simulink model "P2_0D_model_parametrized"  (R2023a)
settings: Solver=ode4  StartTime=0.0  StopTime=inf  FixedStep=Ts  RelTol=1e-3
model workspace (MAT data in the model file):
  Ts : Simulink.Parameter (value not decoded)
undefined symbols (not defined in the file or in its folder): data, HR, left_ventricle_R_wall, MLAP, MRAP, openloop
libraries: Vessel x42, simulink x2
(part 2 of 2)

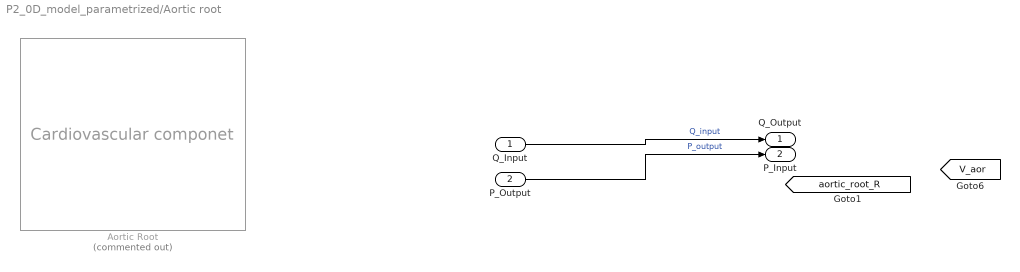
== system P2_0D_model_parametrized/Aortic root ==
  Q_Input : Inport
  P_Output : Inport  Port=2
  Aortic Root : Vessel/Cardiovascular componet  Commented=on  choice=Vessel compartment (L-non-inverted element)  control=None  Y_control=Systemic Arteries  l=aortic_root_l0  r=aortic_root_r0  h=aortic_root_h  n=aortic_root_n  P0=aortic_root_P0  Y=Y_aorta  SI=0  V_tot=V_tot  p_th_on_off=on
      link override "Capillaries (L-non-inverted-element)/ ": GotoTag=pupo
      settings: SourceProductName=CVM
  "Q_Output " : Outport
  "P_Input " : Outport  Port=2
  tag scope: V_aor=global, aortic_root_R=global
  wires:
  P_Output/1 -> "P_Input "/1  "P_output"
  Q_Input/1 -> "Q_Output "/1  "Q_input"

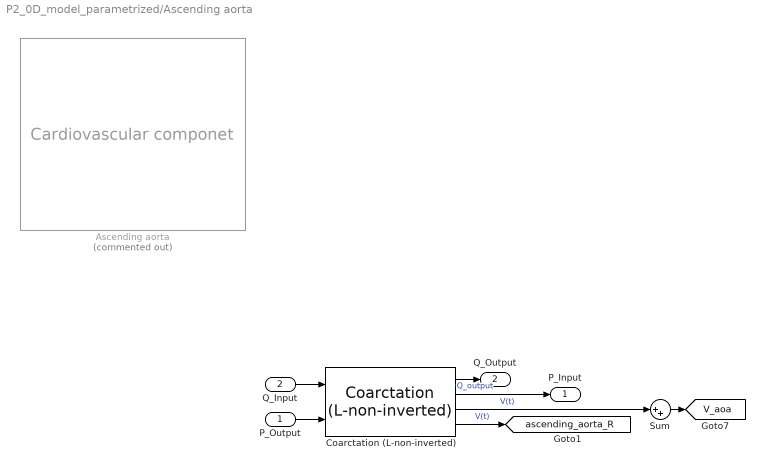
== system P2_0D_model_parametrized/Ascending aorta ==
  P_Output : Inport
  Q_Input : Inport  Port=2
  Ascending aorta : Vessel/Cardiovascular componet  Commented=on  choice=Vessel compartment (L-non-inverted element)  control=None  Y_control=Systemic Arteries  l=ascending_aorta_l0  r=ascending_aorta_r0  h=ascending_aorta_h  n=ascending_aorta_n  P0=ascending_aorta_P0  Y=Y_aorta  SI=0  V_tot=V_tot  p_th_on_off=on
      link override "Capillaries (L-non-inverted-element)/ ": GotoTag=pupo
      settings: SourceProductName=CVM
  Coarctation (L-non-inverted) : Vessel/Coarctation (L-non-inverted)  l=data.vessels{1, 1}.vessel_length  SI=data.vessels{1, 1}.zero_d_element_values.stenosis_coefficient  L0=data.vessels{1, 1}.zero_d_element_values.L  P0=100  Y=Y_aorta  Y_control=Systemic Arteries
      settings: SourceProductName=CVM
  Sum : Sum  Inputs=|++
  "P_Input " : Outport
  "Q_Output " : Outport  Port=2
  tag scope: V_aoa=global, ascending_aorta_R=global
  wires:
  P_Output/1 -> Coarctation (L-non-inverted)/2
  Q_Input/1 -> Coarctation (L-non-inverted)/1
  Coarctation (L-non-inverted)/1 -> "Q_Output "/1  "Q_output"
  Coarctation (L-non-inverted)/3 -> Sum/1  "V(t)"
  Coarctation (L-non-inverted)/4 -> [ascending_aorta_R]  "V(t)"
  Sum/1 -> [V_aoa]
  Coarctation (L-non-inverted)/2 -> "P_Input "/1

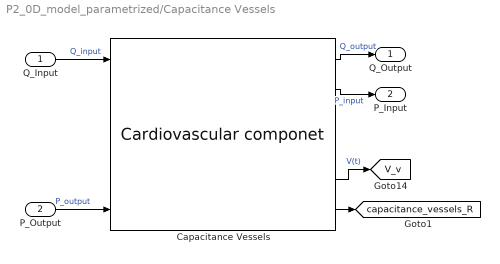
== system P2_0D_model_parametrized/Capacitance Vessels ==
  Q_Input : Inport
  P_Output : Inport  Port=2
  Capacitance Vessels : Vessel/Cardiovascular componet  choice=Vessel compartment (L-non-inverted element)  control=UVV control  Y_control=Systemic Veins  l=capacitance_vessels_l0  r=capacitance_vessels_r0  h=capacitance_vessels_h  n=capacitance_vessels_n  P0=capacitance_vessels_P0  Y=Y_systemic_veins  SI=0  V_tot=V_tot  p_th_on_off=off
      link override "Capillaries (L-non-inverted-element)/ ": GotoTag=pupo
      link override Vessel (L-non-inverted) /Constant1: Value=V0
      link override Vessel (L-non-inverted) Volume control/Constant1: Value=V0
      settings: SourceProductName=CVM
  "Q_Output " : Outport
  "P_Input " : Outport  Port=2
  tag scope: V_v=global, capacitance_vessels_R=global
  wires:
  Capacitance Vessels/5 -> [V_v]  "V(t)"
  Capacitance Vessels/2 -> "P_Input "/1  "P_input"
  P_Output/1 -> Capacitance Vessels/4  "P_output"
  Q_Input/1 -> Capacitance Vessels/1  "Q_input"
  Capacitance Vessels/1 -> "Q_Output "/1  "Q_output"
  Capacitance Vessels/6 -> [capacitance_vessels_R]

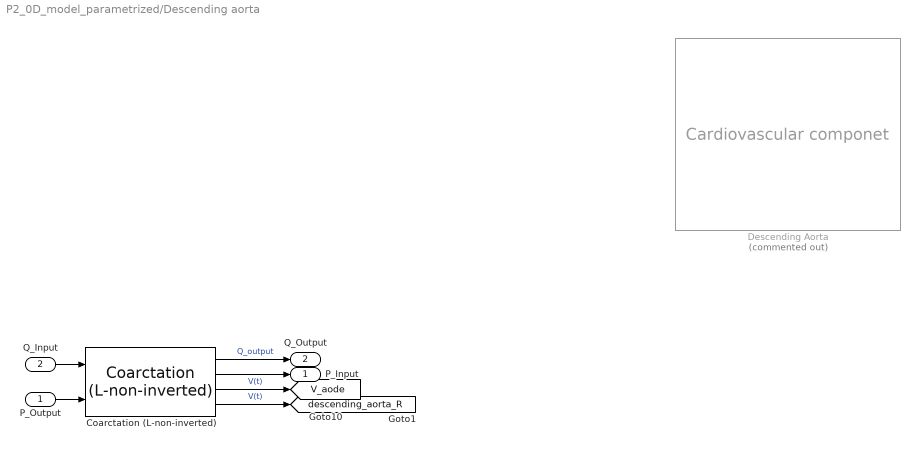
== system P2_0D_model_parametrized/Descending aorta ==
  P_Output : Inport
  Q_Input : Inport  Port=2
  Coarctation (L-non-inverted) : Vessel/Coarctation (L-non-inverted)  l=data.vessels{9,1}.vessel_length  SI=data.vessels{9, 1}.zero_d_element_values.stenosis_coefficient  L0=data.vessels{9, 1}.zero_d_element_values.L  P0=100  Y=Y_aorta  Y_control=Systemic Arteries
      settings: SourceProductName=CVM
  Descending Aorta : Vessel/Cardiovascular componet  Commented=on  choice=Vessel compartment (L-non-inverted element)  control=None  Y_control=Systemic Arteries  l=descending_aorta_l0  r=descending_aorta_r0  h=descending_aorta_h  n=descending_aorta_n  P0=descending_aorta_P0  Y=Y_aorta  SI=0  V_tot=V_tot  p_th_on_off=on
      link override "Capillaries (L-non-inverted-element)/ ": GotoTag=pupo
      settings: SourceProductName=CVM
  "P_Input " : Outport
  "Q_Output " : Outport  Port=2
  tag scope: V_aode=global, descending_aorta_R=global
  wires:
  Coarctation (L-non-inverted)/2 -> "P_Input "/1
  Q_Input/1 -> Coarctation (L-non-inverted)/1
  P_Output/1 -> Coarctation (L-non-inverted)/2
  Coarctation (L-non-inverted)/1 -> "Q_Output "/1  "Q_output"
  Coarctation (L-non-inverted)/3 -> [V_aode]  "V(t)"
  Coarctation (L-non-inverted)/4 -> [descending_aorta_R]  "V(t)"

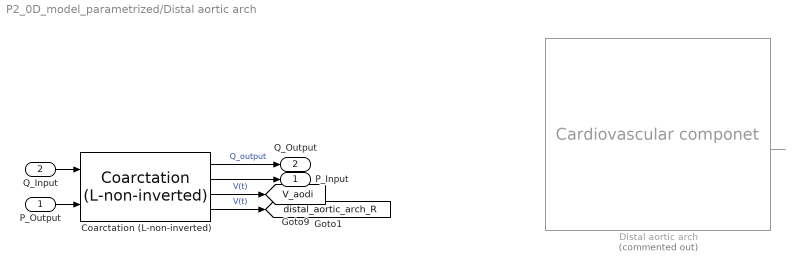
== system P2_0D_model_parametrized/Distal aortic arch ==
  P_Output : Inport
  Q_Input : Inport  Port=2
  Coarctation (L-non-inverted) : Vessel/Coarctation (L-non-inverted)  l=data.vessels{8, 1}.vessel_length  SI=data.vessels{8, 1}.zero_d_element_values.stenosis_coefficient  L0=data.vessels{8, 1}.zero_d_element_values.L  P0=100  Y=Y_aorta  Y_control=Systemic Arteries
      settings: SourceProductName=CVM
  Distal aortic arch : Vessel/Cardiovascular componet  Commented=on  choice=Vessel compartment (L-non-inverted element)  control=None  Y_control=Systemic Arteries  l=distal_aortic_arch_l0  r=distal_aortic_arch_r0  h=distal_aortic_arch_h  n=distal_aortic_arch_n  P0=distal_aortic_arch_P0  Y=Y_aorta  SI=0  V_tot=V_tot  p_th_on_off=on
      link override "Capillaries (L-non-inverted-element)/ ": GotoTag=pupo
      settings: SourceProductName=CVM
  "P_Input " : Outport
  "Q_Output " : Outport  Port=2
  tag scope: V_aodi=global, distal_aortic_arch_R=global
  wires:
  Q_Input/1 -> Coarctation (L-non-inverted)/1
  P_Output/1 -> Coarctation (L-non-inverted)/2
  Distal aortic arch/4 -> ?
  Coarctation (L-non-inverted)/1 -> "Q_Output "/1  "Q_output"
  Coarctation (L-non-inverted)/2 -> "P_Input "/1
  Coarctation (L-non-inverted)/3 -> [V_aodi]  "V(t)"
  Coarctation (L-non-inverted)/4 -> [distal_aortic_arch_R]  "V(t)"

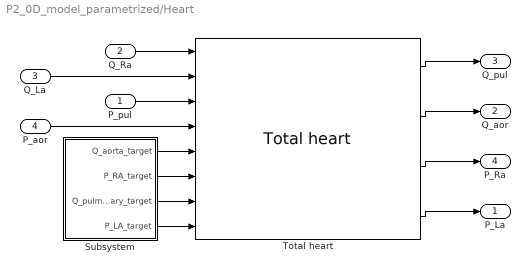
== system P2_0D_model_parametrized/Heart ==
  P_pul : Inport
  Q_Ra : Inport  Port=2
  Q_La : Inport  Port=3
  P_aor : Inport  Port=4
  Subsystem : Subsystem
  Total heart : Vessel/Total heart  BSA=BSA  T0=60/HR  R_lca=left_coronary_artery_R0  R_rca=right_coronary_artery_R0  p_septum_on_off=on  E_max_ra=right_atrium_E_max  E_max_rv=right_ventricle_E_max  E_max_la=left_atrium_E_max  E_max_lv=left_ventricle_E_max  E_min_ra=right_atrium_E_min  E_min_rv=right_ventricle_E_min  E_min_la=left_atrium_E_min  E_min_lv=left_ventricle_E_min  alpha1_ra=right_atrium_alpha1  alpha1_rv=right_ventricle_alpha1  alpha1_la=left_atrium_alpha1  alpha1_lv=left_ventricle_alpha1  alpha2_ra=right_atrium_alpha2  alpha2_rv=right_ventricle_alpha2  alpha2_la=left_atrium_alpha2  alpha2_lv=left_ventricle_alpha2  m1_ra=right_atrium_m1  m1_rv=right_ventricle_m1  m1_la=left_atrium_m1  m1_lv=left_ventricle_m1  m2_ra=right_atrium_m2  m2_rv=right_ventricle_m2  m2_la=left_atrium_m2  m2_lv=left_ventricle_m2  R_wall_ra=right_atrium_R_wall  R_wall_rv=right_ventricle_R_wall  R_wall_la=left_atrium_R_wall  R_wall_lv=left_ventricle_R_wall*1  t_delay_ra=right_atrium_t_delay  t_delay_rv=right_ventricle_t_delay  t_delay_la=left_atrium_t_delay  t_delay_lv=left_ventricle_t_delay  V_0_ra=right_atrium_V0  V_0_rv=right_ventricle_V0  V_0_la=left_atrium_V0  V_0_lv=left_ventricle_V0  v_o_ra=right_atrium_v0  v_o_rv=right_ventricle_v0  v_o_la=left_atrium_v0  v_o_lv=left_ventricle_v0  sigma_ra=right_atrium_sigma  sigma_rv=right_ventricle_sigma  sigma_la=left_atrium_sigma  sigma_lv=left_ventricle_sigma  V_max_ra=right_atrium_V_max  V_max_rv=right_ventricle_V_max  V_max_la=left_atrium_V_max  V_max_lv=left_ventricle_V_max  Q_max_ra=right_atrium_Q_max  Q_max_rv=right_ventricle_Q_max  Q_max_la=left_atrium_Q_max  Q_max_lv=left_ventricle_Q_max  A_ann_tri=tricuspid_valve_A_ann  A_ann_pul=pulmonary_valve_A_ann  A_ann_mit=mitral_valve_A_ann  A_ann_aor=aortic_valve_A_ann  K_vo_tri=tricuspid_valve_K_vo  K_vo_pul=pulmonary_valve_K_vo  K_vo_mit=mitral_valve_K_vo  K_vo_aor=aortic_valve_K_vo  K_vc_tri=tricuspid_valve_K_vc  K_vc_pul=pulmonary_valve_K_vc  K_vc_mit=mitral_valve_K_vc  K_vc_aor=aortic_valve_K_vc  M_st_tri=tricuspid_valve_M_st  M_st_pul=pulmonary_valve_M_st  M_st_mit=mitral_valve_M_st  M_st_aor=aortic_valve_M_st  M_rg_tri=tricuspid_valve_M_rg  M_rg_pul=pulmonary_valve_M_rg  M_rg_mit=mitral_valve_M_rg  M_rg_aor=aortic_valve_M_rg  DP_open_tri=tricuspid_valve_DP_open  DP_open_pul=pulmonary_valve_DP_open  DP_open_mit=mitral_valve_DP_open  DP_open_aor=aortic_valve_DP_open  DP_close_tri=tricuspid_valve_DP_close  DP_close_pul=pulmonary_valve_DP_close  DP_close_mit=mitral_valve_DP_close  DP_close_aor=aortic_valve_DP_close  P_pc_0=P_pc0  K_pc=K_pc  V_pc_0=V_pc  V_pe=PFV  phi_pc=phi_pc  E_sa_0=E_sa0  E_sv_0=E_sv0
      link override Aortic Valve/Saturation1: UpperLimit=100  LowerLimit=0.000
      link override Aortic Valve/Saturation2: UpperLimit=100
      link override Left Atrium: control=Left Atrium
      link override Mitral valve/Saturation1: LowerLimit=0.0000
      link override Pulmonary Valve/Saturation1: UpperLimit=100  LowerLimit=0.0000
      link override Right Atrium: control=Right Atrium
      link override Right Ventricle: control=Right Ventricle
      link override Tricuspid Valve/Saturation1: LowerLimit=0.0000
      link override Volume Control: V_tot_0=V_tot
      settings: SourceProductName=CVM
  P_La : Outport
  Q_aor : Outport  Port=2
  Q_pul : Outport  Port=3
  P_Ra : Outport  Port=4
  wires:
  Total heart/4 -> P_La/1
  Total heart/2 -> Q_aor/1
  Total heart/1 -> Q_pul/1
  Q_Ra/1 -> Total heart/1
  P_pul/1 -> Total heart/3
  Q_La/1 -> Total heart/2
  P_aor/1 -> Total heart/4
  Total heart/3 -> P_Ra/1
  Subsystem/1(Q_aorta_target) -> Total heart/5
  Subsystem/2(P_RA_target) -> Total heart/6
  Subsystem/3(Q_pulmonary_target) -> Total heart/7
  Subsystem/4(P_LA_target) -> Total heart/8

== system P2_0D_model_parametrized/Inferior Caval Vein ==
  Q_Input : Inport
  P_Output : Inport  Port=2
  Inferior Caval Vein : Vessel/Cardiovascular componet  choice=Vessel compartment (L-non-inverted element)  control=None  Y_control=Systemic Veins  l=inferior_caval_vein_l0  r=inferior_caval_vein_r0  h=inferior_caval_vein_h  n=inferior_caval_vein_n  P0=inferior_caval_vein_P0  Y=Y_systemic_veins  SI=0  V_tot=V_tot  p_th_on_off=off
      link override "Capillaries (L-non-inverted-element)/ ": GotoTag=pupo
      settings: SourceProductName=CVM
  "P_Input " : Outport
  "Q_Output " : Outport  Port=2
  tag scope: V_vci=global, inferior_caval_vein_R=global
  wires:
  Inferior Caval Vein/2 -> "P_Input "/1
  Inferior Caval Vein/5 -> [V_vci]
  P_Output/1 -> Inferior Caval Vein/4
  Inferior Caval Vein/1 -> "Q_Output "/1
  Q_Input/1 -> Inferior Caval Vein/1
  Inferior Caval Vein/6 -> [inferior_caval_vein_R]

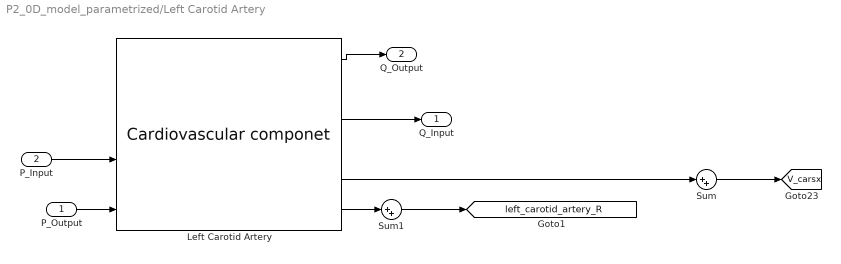
== system P2_0D_model_parametrized/Left Carotid Artery ==
  P_Output : Inport
  P_Input : Inport  Port=2
  Left Carotid Artery : Vessel/Cardiovascular componet  choice=Carotid Artery (L-non-inverted)  control=None  Y_control=Systemic Arteries  l=left_carotid_artery_l0  r=left_carotid_artery_r0  h=left_carotid_artery_h  n=left_carotid_artery_n  P0=left_carotid_artery_P0  Y=Y_aorta  SI=data.vessels{3, 1}.zero_d_element_values.stenosis_coefficient  V_tot=V_tot  p_th_on_off=off
      link override "Capillaries (L-non-inverted-element)/ ": GotoTag=pupo
      settings: SourceProductName=CVM
  Sum : Sum  Inputs=|++
  Sum1 : Sum  Inputs=|++
  Q_Input : Outport
  Q_Output : Outport  Port=2
  tag scope: V_carsx=global, left_carotid_artery_R=global
  wires:
  Left Carotid Artery/5 -> Sum/1
  P_Output/1 -> Left Carotid Artery/4
  Left Carotid Artery/1 -> Q_Output/1
  Sum/1 -> [V_carsx]
  P_Input/1 -> Left Carotid Artery/3
  Sum1/1 -> [left_carotid_artery_R]
  Left Carotid Artery/6 -> Sum1/1
  Left Carotid Artery/3 -> Q_Input/1

== system P2_0D_model_parametrized/Left Carotid Capillaries ==
  P_Output : Inport
  Q_Input : Inport  Port=2
  Left Carotid Capillaries : Vessel/Cardiovascular componet  choice=Capillary compartment (L-non-inverted element)  control=None  Y_control=Systemic Veins  l=left_carotid_capillaries_l0  r=left_carotid_capillaries_r0  h=left_carotid_capillaries_h  n=left_carotid_capillaries_n  P0=left_carotid_capillaries_P0  Y=Y_systemic_veins  SI=0  V_tot=V_tot  p_th_on_off=off
      link override "Capillaries (L-non-inverted-element)/ ": GotoTag=pupo
      settings: SourceProductName=CVM
  P_input : Outport
  Q_Out : Outport  Port=2
  tag scope: V_ccarsx=global, left_carotid_capillaries_R=global
  wires:
  Left Carotid Capillaries/5 -> [V_ccarsx]
  P_Output/1 -> Left Carotid Capillaries/4
  Left Carotid Capillaries/1 -> Q_Out/1
  Left Carotid Capillaries/2 -> P_input/1
  Q_Input/1 -> Left Carotid Capillaries/1
  Left Carotid Capillaries/6 -> [left_carotid_capillaries_R]

== system P2_0D_model_parametrized/Left Carotid Resistance Artery ==
  P_Output : Inport
  Q_Input1 : Inport  Port=2
  Left Carotid Resistance Artery : Vessel/Cardiovascular componet  choice=Vessel compartment (L-non-inverted element)  control=SVR control  Y_control=Systemic Arteries  l=left_carotid_resistance_artery_l0  r=left_carotid_resistance_artery_r0  h=left_carotid_resistance_artery_h  n=left_carotid_resistance_artery_n  P0=left_carotid_resistance_artery_P0  Y=Y_aorta  SI=0  V_tot=V_tot  p_th_on_off=off
      link override "Capillaries (L-non-inverted-element)/ ": GotoTag=pupo
      settings: SourceProductName=CVM
  P_input : Outport
  Q_Output : Outport  Port=2
  tag scope: V_rcarsx=global, left_carotid_resistance_artery_R=global
  wires:
  Left Carotid Resistance Artery/5 -> [V_rcarsx]
  Left Carotid Resistance Artery/1 -> Q_Output/1
  Q_Input1/1 -> Left Carotid Resistance Artery/1
  Left Carotid Resistance Artery/2 -> P_input/1
  P_Output/1 -> Left Carotid Resistance Artery/4
  Left Carotid Resistance Artery/6 -> [left_carotid_resistance_artery_R]

== system P2_0D_model_parametrized/Left Carotid Vein ==
  P_Output : Inport
  Q_Input : Inport  Port=2
  Left Carotid Vein : Vessel/Cardiovascular componet  choice=Vessel compartment (L-non-inverted element)  control=UVV control  Y_control=Systemic Veins  l=left_carotid_vein_l0  r=left_carotid_vein_r0  h=left_carotid_vein_h  n=left_carotid_vein_n  P0=left_carotid_vein_P0  Y=Y_systemic_veins  SI=0  V_tot=V_tot  p_th_on_off=off
      link override "Capillaries (L-non-inverted-element)/ ": GotoTag=pupo
      settings: SourceProductName=CVM
  "P_Input " : Outport
  "Q_Output " : Outport  Port=2
  tag scope: V_vcarsx=global, left_carotid_vein_R=global
  wires:
  Left Carotid Vein/5 -> [V_vcarsx]
  P_Output/1 -> Left Carotid Vein/4
  Left Carotid Vein/2 -> "P_Input "/1
  Q_Input/1 -> Left Carotid Vein/1
  Left Carotid Vein/1 -> "Q_Output "/1
  Left Carotid Vein/6 -> [left_carotid_vein_R]

== system P2_0D_model_parametrized/Peripheral Arteries ==
  P_Output : Inport
  Q_Input : Inport  Port=2
  Peripheral Arteries : Vessel/Cardiovascular componet  choice=Vessel compartment (L-non-inverted element)  control=SVR control  Y_control=Systemic Arteries  l=peripheral_arteries_l0  r=peripheral_arteries_r0  h=peripheral_arteries_h  n=peripheral_arteries_n  P0=peripheral_arteries_P0  Y=Y_aorta  SI=0  V_tot=V_tot  p_th_on_off=off
      link override "Capillaries (L-non-inverted-element)/ ": GotoTag=pupo
      settings: SourceProductName=CVM
  "P_Input " : Outport
  "Q_Output " : Outport  Port=2
  tag scope: V_a=global, peripheral_arteries_R=global
  wires:
  Peripheral Arteries/5 -> [V_a]
  Peripheral Arteries/2 -> "P_Input "/1
  P_Output/1 -> Peripheral Arteries/4
  Q_Input/1 -> Peripheral Arteries/1
  Peripheral Arteries/1 -> "Q_Output "/1
  Peripheral Arteries/6 -> [peripheral_arteries_R]

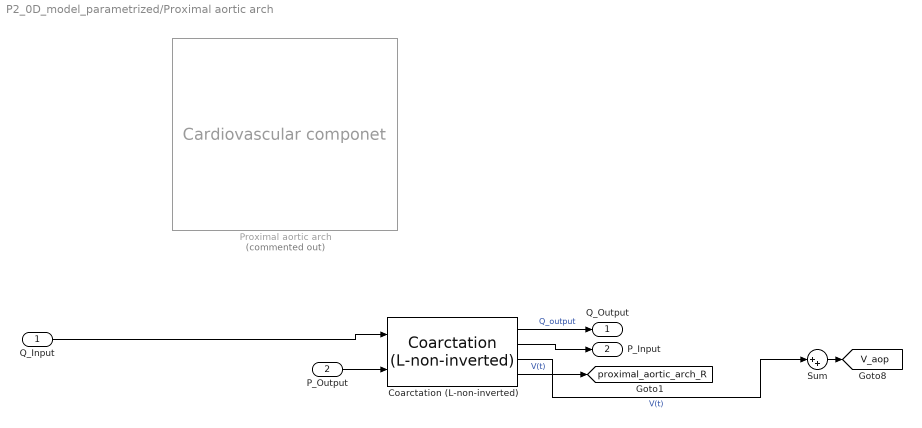
== system P2_0D_model_parametrized/Proximal aortic arch ==
  Q_Input : Inport
  P_Output : Inport  Port=2
  Coarctation (L-non-inverted) : Vessel/Coarctation (L-non-inverted)  l=data.vessels{7, 1}.vessel_length  SI=data.vessels{7, 1}.zero_d_element_values.stenosis_coefficient  L0=data.vessels{7, 1}.zero_d_element_values.L  P0=100  Y=Y_aorta  Y_control=Systemic Arteries
      settings: SourceProductName=CVM
  Proximal aortic arch : Vessel/Cardiovascular componet  Commented=on  choice=Vessel compartment (L-non-inverted element)  control=None  Y_control=Systemic Arteries  l=proximal_aortic_arch_l0  r=proximal_aortic_arch_r0  h=proximal_aortic_arch_h  n=proximal_aortic_arch_n  P0=proximal_aortic_arch_P0  Y=Y_aorta  SI=0  V_tot=V_tot  p_th_on_off=on
      link override "Capillaries (L-non-inverted-element)/ ": GotoTag=pupo
      settings: SourceProductName=CVM
  Sum : Sum  Inputs=|++
  "Q_Output " : Outport
  "P_Input " : Outport  Port=2
  tag scope: V_aop=global, proximal_aortic_arch_R=global
  wires:
  P_Output/1 -> Coarctation (L-non-inverted)/2
  Q_Input/1 -> Coarctation (L-non-inverted)/1
  Coarctation (L-non-inverted)/3 -> Sum/1  "V(t)"
  Coarctation (L-non-inverted)/4 -> [proximal_aortic_arch_R]  "V(t)"
  Coarctation (L-non-inverted)/1 -> "Q_Output "/1  "Q_output"
  Sum/1 -> [V_aop]
  Coarctation (L-non-inverted)/2 -> "P_Input "/1

== system P2_0D_model_parametrized/Pulmonary Arteries ==
  Q_Input : Inport
  P_Output : Inport  Port=2
  Pulmonary Arteries : Vessel/Cardiovascular componet  choice=Vessel compartment (L-non-inverted element)  control=None  Y_control=Pulmonary Arteries  l=pulmonary_arteries_l0  r=pulmonary_arteries_r0  h=pulmonary_arteries_h  n=pulmonary_arteries_n  P0=pulmonary_arteries_P0  Y=Y_pulmonary_arteries  SI=0  V_tot=V_tot  p_th_on_off=on
      link override "Capillaries (L-non-inverted-element)/ ": GotoTag=pupo
      settings: SourceProductName=CVM
  "Q_Output " : Outport
  "P_Input " : Outport  Port=2
  tag scope: V_pua=global, pulmonary_arteries_R=global
  wires:
  Pulmonary Arteries/5 -> [V_pua]
  Pulmonary Arteries/1 -> "Q_Output "/1
  Pulmonary Arteries/2 -> "P_Input "/1
  P_Output/1 -> Pulmonary Arteries/4
  Q_Input/1 -> Pulmonary Arteries/1
  Pulmonary Arteries/6 -> [pulmonary_arteries_R]

== system P2_0D_model_parametrized/Pulmonary Capillaries ==
  Q_Input : Inport
  P_Output : Inport  Port=2
  Pulmonary Capillaries : Vessel/Cardiovascular componet  choice=Capillary compartment (L-non-inverted element)  control=PVR control  Y_control=Pulmonary Veins  l=pulmonary_capillaries_l0  r=pulmonary_capillaries_r0  h=pulmonary_capillaries_h  n=pulmonary_capillaries_n  P0=pulmonary_capillaries_P0  Y=Y_pulmonary_veins  SI=0  V_tot=V_tot  p_th_on_off=on
      link override "Capillaries (L-non-inverted-element)/ ": GotoTag=pupo
      settings: SourceProductName=CVM
  "Q_Output " : Outport
  "P_Input " : Outport  Port=2
  tag scope: V_puc=global, pulmonary_capillaries_R=global
  wires:
  Pulmonary Capillaries/5 -> [V_puc]
  Pulmonary Capillaries/1 -> "Q_Output "/1
  Pulmonary Capillaries/2 -> "P_Input "/1
  P_Output/1 -> Pulmonary Capillaries/4
  Q_Input/1 -> Pulmonary Capillaries/1
  Pulmonary Capillaries/6 -> [pulmonary_capillaries_R]

== system P2_0D_model_parametrized/Pulmonary Resistance Arteries ==
  Q_Input : Inport
  P_Output : Inport  Port=2
  Pulmonary Resistance Arteries : Vessel/Cardiovascular componet  choice=Vessel compartment (L-non-inverted element)  control=PVR control  Y_control=Pulmonary Veins  l=pulmonary_resistance_arteries_l0  r=pulmonary_resistance_arteries_r0  h=pulmonary_resistance_arteries_h  n=pulmonary_resistance_arteries_n  P0=pulmonary_resistance_arteries_P0  Y=Y_pulmonary_veins  SI=0  V_tot=V_tot  p_th_on_off=on
      link override "Capillaries (L-non-inverted-element)/ ": GotoTag=pupo
      settings: SourceProductName=CVM
  "Q_Output " : Outport
  "P_Input " : Outport  Port=2
  tag scope: V_pur=global, pulmonary_resistance_arteries_R=global
  wires:
  Pulmonary Resistance Arteries/5 -> [V_pur]
  Pulmonary Resistance Arteries/2 -> "P_Input "/1
  P_Output/1 -> Pulmonary Resistance Arteries/4
  Pulmonary Resistance Arteries/1 -> "Q_Output "/1
  Q_Input/1 -> Pulmonary Resistance Arteries/1
  Pulmonary Resistance Arteries/6 -> [pulmonary_resistance_arteries_R]

== system P2_0D_model_parametrized/Pulmonary Small Veins ==
  Q_Input : Inport
  P_Output : Inport  Port=2
  Pulmonary Small Veins : Vessel/Cardiovascular componet  choice=Vessel compartment (L-non-inverted element)  control=PVR control  Y_control=Pulmonary Veins  l=pulmonary_small_veins_l0  r=pulmonary_small_veins_r0  h=pulmonary_small_veins_h  n=pulmonary_small_veins_n  P0=pulmonary_small_veins_P0  Y=Y_pulmonary_veins  SI=0  V_tot=V_tot  p_th_on_off=on
      link override "Capillaries (L-non-inverted-element)/ ": GotoTag=pupo
      settings: SourceProductName=CVM
  "Q_Output " : Outport
  "P_Input " : Outport  Port=2
  tag scope: V_pusv=global, pulmonary_small_veins_R=global
  wires:
  Pulmonary Small Veins/5 -> [V_pusv]
  Pulmonary Small Veins/1 -> "Q_Output "/1
  Q_Input/1 -> Pulmonary Small Veins/1
  Pulmonary Small Veins/2 -> "P_Input "/1
  P_Output/1 -> Pulmonary Small Veins/4
  Pulmonary Small Veins/6 -> [pulmonary_small_veins_R]

== system P2_0D_model_parametrized/Pulmonary Trunk ==
  P_Output : Inport
  Q_Input : Inport  Port=2
  Pulmonary Trunk : Vessel/Cardiovascular componet  choice=Vessel compartment (L-non-inverted element)  control=None  Y_control=Pulmonary Arteries  l=pulmonary_trunk_l0  r=pulmonary_trunk_r0  h=pulmonary_trunk_h  n=pulmonary_trunk_n  P0=pulmonary_trunk_P0  Y=Y_pulmonary_arteries  SI=0  V_tot=V_tot  p_th_on_off=on
      link override "Capillaries (L-non-inverted-element)/ ": GotoTag=pupo
      settings: SourceProductName=CVM
  "P_Input " : Outport
  "Q_Output " : Outport  Port=2
  tag scope: V_put=global, pulmonary_trunk_R=global
  wires:
  Pulmonary Trunk/2 -> "P_Input "/1
  Pulmonary Trunk/1 -> "Q_Output "/1
  P_Output/1 -> Pulmonary Trunk/4
  Pulmonary Trunk/5 -> [V_put]
  Q_Input/1 -> Pulmonary Trunk/1
  Pulmonary Trunk/6 -> [pulmonary_trunk_R]

== system P2_0D_model_parametrized/Pulmonary Veins ==
  Q_Input : Inport
  P_Output : Inport  Port=2
  Pulmonary Veins : Vessel/Cardiovascular componet  choice=Vessel compartment (L-non-inverted element)  control=None  Y_control=Pulmonary Veins  l=pulmonary_veins_l0  r=pulmonary_veins_r0  h=pulmonary_veins_h  n=pulmonary_veins_n  P0=pulmonary_veins_P0  Y=Y_pulmonary_veins  SI=0  V_tot=V_tot  p_th_on_off=on
      link override "Capillaries (L-non-inverted-element)/ ": GotoTag=pupo
      settings: SourceProductName=CVM
  "Q_Output " : Outport
  "P_Input " : Outport  Port=2
  tag scope: V_puv=global, pulmonary_veins_R=global
  wires:
  Pulmonary Veins/2 -> "P_Input "/1
  Pulmonary Veins/1 -> "Q_Output "/1
  Pulmonary Veins/5 -> [V_puv]
  P_Output/1 -> Pulmonary Veins/4
  Q_Input/1 -> Pulmonary Veins/1
  Pulmonary Veins/6 -> [pulmonary_veins_R]

== system P2_0D_model_parametrized/Resistance Arteries ==
  Q_Input : Inport
  P_Output : Inport  Port=2
  Resistance Arteries : Vessel/Cardiovascular componet  choice=Vessel compartment (L-non-inverted element)  control=SVR control  Y_control=Systemic Arteries  l=resistance_arteries_l0  r=resistance_arteries_r0  h=resistance_arteries_h  n=resistance_arteries_n  P0=resistance_arteries_P0  Y=Y_aorta  SI=0  V_tot=V_tot  p_th_on_off=off
      link override "Capillaries (L-non-inverted-element)/ ": GotoTag=pupo
      settings: SourceProductName=CVM
  "Q_Output " : Outport
  "P_Input " : Outport  Port=2
  tag scope: V_r=global, resistance_arteries_R=global
  wires:
  Resistance Arteries/5 -> [V_r]
  Resistance Arteries/1 -> "Q_Output "/1
  Resistance Arteries/2 -> "P_Input "/1
  P_Output/1 -> Resistance Arteries/4
  Q_Input/1 -> Resistance Arteries/1
  Resistance Arteries/6 -> [resistance_arteries_R]

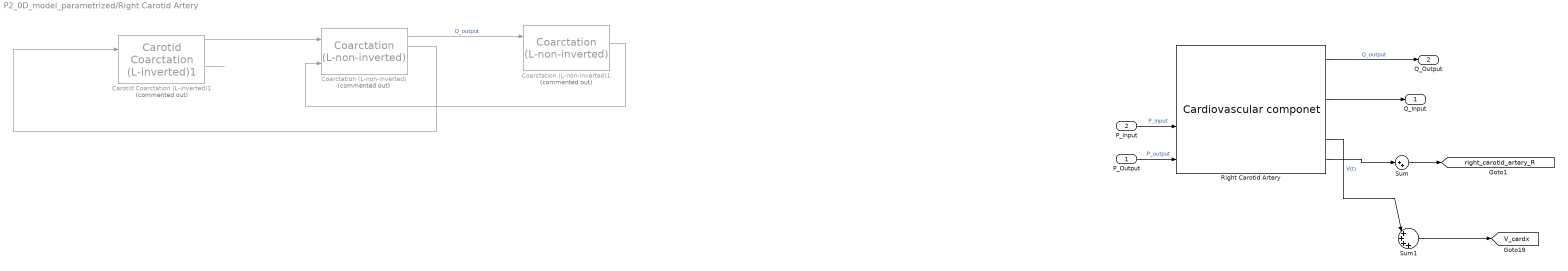
== system P2_0D_model_parametrized/Right Carotid Artery ==
  P_Output : Inport
  P_Input : Inport  Port=2
  Carotid Coarctation (L-inverted)1 : Vessel/Carotid Coarctation (L-inverted)1  Commented=on  l=data.vessels{10, 1}.vessel_length  SI=data.vessels{10, 1}.zero_d_element_values.stenosis_coefficient  L0=data.vessels{10, 1}.zero_d_element_values.L  P0=100  Y=Y_aorta  Y_control=Systemic arteries
      settings: SourceProductName=CVM
  Coarctation (L-non-inverted) : Vessel/Coarctation (L-non-inverted)  Commented=on  l=data.vessels{11, 1}.vessel_length  SI=data.vessels{11, 1}.zero_d_element_values.stenosis_coefficient  L0=data.vessels{11, 1}.zero_d_element_values.L  P0=100  Y=Y_aorta  Y_control=Systemic Arteries
      settings: SourceProductName=CVM
  Coarctation (L-non-inverted)1 : Vessel/Coarctation (L-non-inverted)  Commented=on  l=data.vessels{12, 1}.vessel_length  SI=data.vessels{12, 1}.zero_d_element_values.stenosis_coefficient  L0=data.vessels{12, 1}.zero_d_element_values.L  P0=100  Y=Y_aorta  Y_control=Systemic Arteries
      settings: SourceProductName=CVM
  Right Carotid Artery : Vessel/Cardiovascular componet  choice=Carotid Artery (L-non-inverted)  control=None  Y_control=Systemic Arteries  l=right_carotid_artery_l0  r=right_carotid_artery_r0  h=right_carotid_artery_h  n=right_carotid_artery_n  P0=right_carotid_artery_P0  Y=Y_aorta  SI=data.vessels{2, 1}.zero_d_element_values.stenosis_coefficient  V_tot=V_tot  p_th_on_off=off
      link override "Capillaries (L-non-inverted-element)/ ": GotoTag=pupo
      settings: SourceProductName=CVM
  Sum : Sum  Inputs=|++
  Sum1 : Sum  Inputs=|++++
  Q_Input : Outport
  Q_Output : Outport  Port=2
  tag scope: V_cardx=global, right_carotid_artery_R=global
  wires:
  P_Output/1 -> Right Carotid Artery/4  "P_output"
  Right Carotid Artery/1 -> Q_Output/1  "Q_output"
  Sum/1 -> [right_carotid_artery_R]
  Sum1/1 -> [V_cardx]
  Right Carotid Artery/3 -> Q_Input/1
  ? -> Carotid Coarctation (L-inverted)1/2  "P_input"
  Carotid Coarctation (L-inverted)1/1 -> Coarctation (L-non-inverted)/1
  Coarctation (L-non-inverted)/1 -> Coarctation (L-non-inverted)1/1  "Q_output"
  Coarctation (L-non-inverted)/2 -> Carotid Coarctation (L-inverted)1/1
  Coarctation (L-non-inverted)1/2 -> Coarctation (L-non-inverted)/2
  Carotid Coarctation (L-inverted)1/3 -> ?
  Right Carotid Artery/6 -> Sum/1
  Right Carotid Artery/5 -> Sum1/1  "V(t)"
  P_Input/1 -> Right Carotid Artery/3  "P_input"

== system P2_0D_model_parametrized/Right Carotid Capillaries ==
  P_Output : Inport
  Q_Input1 : Inport  Port=2
  Right Carotid Capillaries : Vessel/Cardiovascular componet  choice=Capillary compartment (L-non-inverted element)  control=None  Y_control=Systemic Veins  l=right_carotid_capillaries_l0  r=right_carotid_capillaries_r0  h=right_carotid_capillaries_h  n=right_carotid_capillaries_n  P0=right_carotid_capillaries_P0  Y=Y_systemic_veins  SI=0  V_tot=V_tot  p_th_on_off=off
      link override "Capillaries (L-non-inverted-element)/ ": GotoTag=pupo
      settings: SourceProductName=CVM
  P_input : Outport
  Q_Out : Outport  Port=2
  tag scope: V_ccardx=global, right_carotid_capillaries_R=global
  wires:
  Right Carotid Capillaries/5 -> [V_ccardx]
  Right Carotid Capillaries/1 -> Q_Out/1
  P_Output/1 -> Right Carotid Capillaries/4
  Q_Input1/1 -> Right Carotid Capillaries/1
  Right Carotid Capillaries/2 -> P_input/1
  Right Carotid Capillaries/6 -> [right_carotid_capillaries_R]

== system P2_0D_model_parametrized/Right Carotid Resistance Artery ==
  P_Output : Inport
  Q_Input1 : Inport  Port=2
  Right Carotid Resistance Artery : Vessel/Cardiovascular componet  choice=Vessel compartment (L-non-inverted element)  control=SVR control  Y_control=Systemic Arteries  l=right_carotid_resistance_artery_l0  r=right_carotid_resistance_artery_r0  h=right_carotid_resistance_artery_h  n=right_carotid_resistance_artery_n  P0=right_carotid_resistance_artery_P0  Y=Y_aorta  SI=0  V_tot=V_tot  p_th_on_off=off
      link override "Capillaries (L-non-inverted-element)/ ": GotoTag=pupo
      link override Vessel (L-inverted)/IC1: Value=0
      settings: SourceProductName=CVM
  P_input : Outport
  Q_Output : Outport  Port=2
  tag scope: V_rcardx=global, right_carotid_resistance_artery_R=global
  wires:
  Right Carotid Resistance Artery/5 -> [V_rcardx]
  P_Output/1 -> Right Carotid Resistance Artery/4
  Q_Input1/1 -> Right Carotid Resistance Artery/1
  Right Carotid Resistance Artery/2 -> P_input/1
  Right Carotid Resistance Artery/1 -> Q_Output/1
  Right Carotid Resistance Artery/6 -> [right_carotid_resistance_artery_R]

== system P2_0D_model_parametrized/Right Carotid Vein ==
  P_Output : Inport
  Q_Input : Inport  Port=2
  Right Carotid Vein : Vessel/Cardiovascular componet  choice=Vessel compartment (L-non-inverted element)  control=UVV control  Y_control=Systemic Veins  l=right_carotid_vein_l0  r=right_carotid_vein_r0  h=right_carotid_vein_h  n=right_carotid_vein_n  P0=right_carotid_vein_P0  Y=Y_systemic_veins  SI=0  V_tot=V_tot  p_th_on_off=off
      link override "Capillaries (L-non-inverted-element)/ ": GotoTag=pupo
      settings: SourceProductName=CVM
  "P_Input " : Outport
  "Q_Output " : Outport  Port=2
  tag scope: V_vcardx=global, right_carotid_vein_R=global
  wires:
  Right Carotid Vein/5 -> [V_vcardx]
  P_Output/1 -> Right Carotid Vein/4
  Right Carotid Vein/2 -> "P_Input "/1
  Q_Input/1 -> Right Carotid Vein/1
  Right Carotid Vein/1 -> "Q_Output "/1
  Right Carotid Vein/6 -> [right_carotid_vein_R]

== system P2_0D_model_parametrized/Superior Caval Vein ==
  Q_Input : Inport
  P_Output : Inport  Port=2
  Superior Caval Vein : Vessel/Cardiovascular componet  choice=Vessel compartment (L-non-inverted element)  control=None  Y_control=Systemic Veins  l=superior_caval_vein_l0  r=superior_caval_vein_r0  h=superior_caval_vein_h  n=superior_caval_vein_n  P0=superior_caval_vein_P0  Y=Y_systemic_veins  SI=0  V_tot=V_tot  p_th_on_off=off
      link override "Capillaries (L-non-inverted-element)/ ": GotoTag=pupo
      settings: SourceProductName=CVM
  "Q_Output " : Outport
  "P_Input " : Outport  Port=2
  tag scope: V_vcs=global, superior_caval_vein_R=global
  wires:
  Superior Caval Vein/2 -> "P_Input "/1
  Superior Caval Vein/1 -> "Q_Output "/1
  P_Output/1 -> Superior Caval Vein/4
  Superior Caval Vein/5 -> [V_vcs]
  Q_Input/1 -> Superior Caval Vein/1
  Superior Caval Vein/6 -> [superior_caval_vein_R]

== system P2_0D_model_parametrized/Systemic Capillaries  ==
  P_Output : Inport
  Q_Input : Inport  Port=2
  Systemic Capillaries : Vessel/Cardiovascular componet  choice=Capillary compartment (L-non-inverted element)  control=None  Y_control=Systemic Veins  l=systemic_capillaries_l0  r=systemic_capillaries_r0  h=systemic_capillaries_h  n=systemic_capillaries_n  P0=systemic_capillaries_P0  Y=Y_systemic_veins  SI=0  V_tot=V_tot  p_th_on_off=off
      link override "Capillaries (L-non-inverted-element)/ ": GotoTag=pupo
      settings: SourceProductName=CVM
  "P_Input " : Outport
  "Q_Output " : Outport  Port=2
  tag scope: V_c=global, systemic_capillaries_R=global
  wires:
  Systemic Capillaries/5 -> [V_c]  "V(t)"
  Systemic Capillaries/2 -> "P_Input "/1  "P_input"
  P_Output/1 -> Systemic Capillaries/4  "P_output"
  Q_Input/1 -> Systemic Capillaries/1  "Q_input"
  Systemic Capillaries/1 -> "Q_Output "/1  "Q_output"
  Systemic Capillaries/6 -> [systemic_capillaries_R]

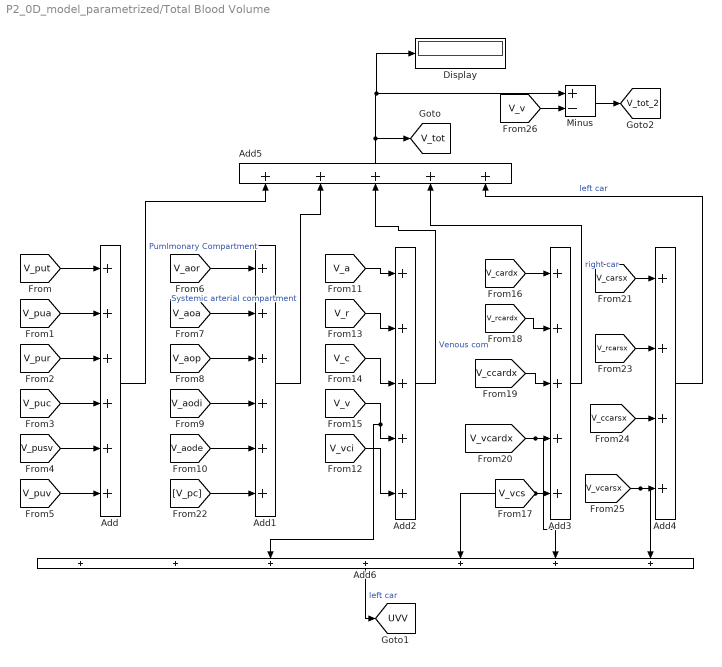
== system P2_0D_model_parametrized/Total Blood Volume ==
  Add : Sum  Inputs=++++++
  Add1 : Sum  Inputs=++++++
  Add2 : Sum  Inputs=+++++
  Add3 : Sum  Inputs=+++++
  Add4 : Sum  Inputs=++++
  Add5 : Sum  Inputs=+++++
  Add6 : Sum  Inputs=+++++++
  Display : Display
  Minus : Sum  Inputs=+-
  tag scope: UVV=global, V_tot=global, V_tot_2=global
  wires:
  [V_put] -> Add/1
  [V_pua] -> Add/2
  [V_pur] -> Add/3
  [V_puc] -> Add/4
  [V_pusv] -> Add/5
  [V_puv] -> Add/6
  [V_aor] -> Add1/1
  [V_aoa] -> Add1/2
  [V_aop] -> Add1/3
  [V_aodi] -> Add1/4
  [V_aode] -> Add1/5
  [V_a] -> Add2/1
  [V_r] -> Add2/2
  [V_c] -> Add2/3
  [V_v] -> Add6/3, Add2/4
  [V_vci] -> Add2/5
  [V_cardx] -> Add3/1
  [V_rcardx] -> Add3/2
  [V_ccardx] -> Add3/3
  [V_vcardx] -> Add6/6, Add3/4
  [V_vcs] -> Add6/5, Add3/5
  [V_carsx] -> Add4/1
  [V_rcarsx] -> Add4/2
  [V_ccarsx] -> Add4/3
  [V_pc] -> Add1/6
  Add/1 -> Add5/1  "Pumlmonary Compartment"
  Add1/1 -> Add5/2  "Systemic arterial compartment"
  Add2/1 -> Add5/3  "Venous com"
  Add3/1 -> Add5/4  "right car"
  Add4/1 -> Add5/5  "left car"
  Add5/1 -> [V_tot], Display/1, Minus/1
  [V_vcarsx] -> Add6/7, Add4/4
  Add6/1 -> [UVV]  "left car"
  Minus/1 -> [V_tot_2]
  [V_v] -> Minus/2

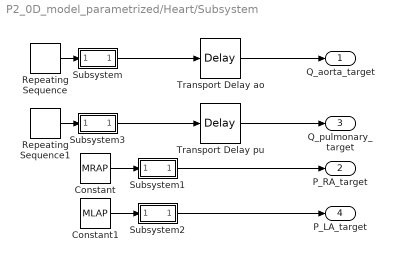
== system P2_0D_model_parametrized/Heart/Subsystem ==
  Constant : Constant  Value=MRAP
  Constant1 : Constant  Value=MLAP
  Repeating Sequence : simulink/Sources/Repeating Sequence  rep_seq_t=t  rep_seq_y=Q
  Repeating Sequence1 : simulink/Sources/Repeating Sequence  rep_seq_t=t  rep_seq_y=Q_p
  Subsystem : Subsystem
  Subsystem1 : Subsystem
  Subsystem2 : Subsystem
  Subsystem3 : Subsystem
  Transport Delay ao : TransportDelay  DelayTime=0
  Transport Delay pu : TransportDelay  DelayTime=0
  Q_aorta_target : Outport
  P_RA_target : Outport  Port=2
  Q_pulmonary_target : Outport  Port=3
  P_LA_target : Outport  Port=4
  wires:
  Repeating Sequence/1 -> Subsystem/1(In1)
  Constant/1 -> Subsystem1/1(In1)
  Constant1/1 -> Subsystem2/1(In1)
  Subsystem1/1(Out1) -> P_RA_target/1
  Subsystem2/1(Out1) -> P_LA_target/1
  Subsystem/1(Q_aorta_target) -> Transport Delay ao/1
  Repeating Sequence1/1 -> Subsystem3/1(In1)
  Subsystem3/1(Q_pulmonary_target) -> Transport Delay pu/1
  Transport Delay ao/1 -> Q_aorta_target/1
  Transport Delay pu/1 -> Q_pulmonary_target/1

== system P2_0D_model_parametrized/Heart/Subsystem/Subsystem ==
  In1 : Inport
  Constant2 : Constant  Value=openloop
  NaN : Constant  Value=NaN  OutDataTypeStr=Inherit: Inherit via back propagation
  Switch : Switch  Criteria=u2 > Threshold  SaturateOnIntegerOverflow=off  InputSameDT=off
  Q_aorta_target : Outport
  wires:
  In1/1 -> Switch/1
  Switch/1 -> Q_aorta_target/1
  Constant2/1 -> Switch/2
  NaN/1 -> Switch/3

== system P2_0D_model_parametrized/Heart/Subsystem/Subsystem1 ==
  In1 : Inport
  Constant2 : Constant  Value=openloop
  NaN : Constant  Value=NaN  OutDataTypeStr=Inherit: Inherit via back propagation
  Switch : Switch  Criteria=u2 > Threshold  SaturateOnIntegerOverflow=off  InputSameDT=off
  Out1 : Outport
  wires:
  NaN/1 -> Switch/3
  Constant2/1 -> Switch/2
  Switch/1 -> Out1/1
  In1/1 -> Switch/1

== system P2_0D_model_parametrized/Heart/Subsystem/Subsystem2 ==
  In1 : Inport
  Constant2 : Constant  Value=openloop
  NaN : Constant  Value=NaN  OutDataTypeStr=Inherit: Inherit via back propagation
  Switch : Switch  Criteria=u2 > Threshold  SaturateOnIntegerOverflow=off  InputSameDT=off
  Out1 : Outport
  wires:
  In1/1 -> Switch/1
  Switch/1 -> Out1/1
  Constant2/1 -> Switch/2
  NaN/1 -> Switch/3

== system P2_0D_model_parametrized/Heart/Subsystem/Subsystem3 ==
  In1 : Inport
  Constant2 : Constant  Value=openloop
  NaN : Constant  Value=NaN  OutDataTypeStr=Inherit: Inherit via back propagation
  Switch : Switch  Criteria=u2 > Threshold  SaturateOnIntegerOverflow=off  InputSameDT=off
  Q_pulmonary_target : Outport
  wires:
  In1/1 -> Switch/1
  Switch/1 -> Q_pulmonary_target/1
  Constant2/1 -> Switch/2
  NaN/1 -> Switch/3
